simulink model "non_Cascaded_I_PD"  (R2025a)
settings: Solver=VariableStepAuto  StartTime=0.0  StopTime=500  FixedStep=0.01  RelTol=1e-3
InitFcn:
  | parameters
values from neighbouring files (symbols this model uses):
  A = pi*(d/2)^2    (= 0.00321699087728)    [parameters.m]    (also in simulations_code.m = 0.00785398163397; test.m = 0.00785398163397)
  A_cross = 0.090    (= 0.09)    [parameters.m]    (also in simulations_code.m = 0.07; test.m = 0.07)
  C_d = 0.136    [parameters.m]    (also in simulations_code.m = 1; test.m = 1)
  constant_amplitude = 0    [Mission.m]    (also in sensitivity.m)
  d1 = 2    [parameters.m]    (also in simulation_matlab.m = 5; simulations_code.m = 5; test.m = 5)
  F_pos = 0.300 * g + m*g    (= 49.70727)    [parameters.m]    (also in sensitivity.m = 0.300 * g + m_values(i)*g; simulation_matlab.m = 2.94; simulations_code.m = 32.37; test.m = 32.37)
  g = 9.81    [parameters.m]    (also in simulation_matlab.m; simulations_code.m; test.m)
  k_m = 50    [simulation_matlab.m]    (also in simulations_code.m = 5; test.m = 5)
  m = 4.567+0.2    (= 4.767)    [parameters.m]    (also in simulation_matlab.m = 3; simulations_code.m = 3; test.m = 3)
  m_a = 0    [parameters.m]    (also in simulation_matlab.m; simulations_code.m = 2.5; test.m = 2.5)
  p = 0.002    [parameters.m]    (also in simulation_matlab.m; simulations_code.m; test.m)
  rho = 1000    [parameters.m]    (also in simulation_matlab.m; simulations_code.m; test.m)
  sine_amplitude = 0    [Mission.m]    (also in sensitivity.m)
  x_max = V_max / A    (= 0.155424749113)    [parameters.m]    (also in simulations_code.m = 0.0636619772368)
  z_ref = 3    [compare_controllers.m]    (also in simulation_matlab.m = 5; simulations_code.m; test.m; test_scenarios.m = 5)
libraries: slpidlib x1
settings Model: Creator=hannasennero  LastModifiedBy=hannasennero
settings SolverCC: ZeroCrossAlgorithm=Adaptive
settings DebuggingCC: IgnoredZcDiagnostic=none

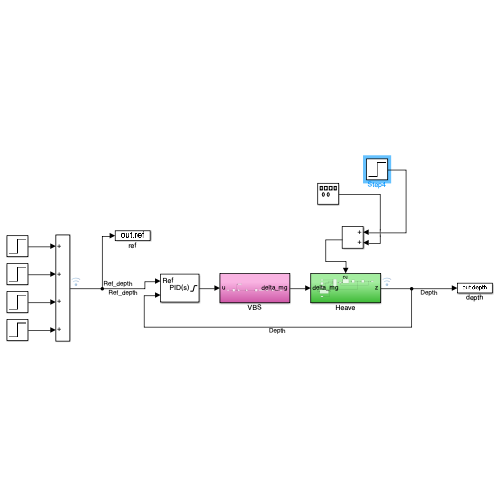
[thumbnail: Simulink's stored preview of the top-level diagram]
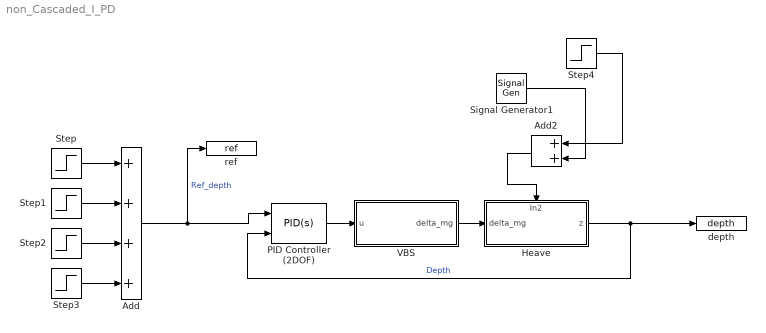
== system non_Cascaded_I_PD ==
  Add : Sum  Inputs=++++
  Add2 : Sum
  Heave : Subsystem
      settings: PortSchema="{\"entries\":[{\"content\":{\"sides\":[{\"content\":{\"connectorIds\":[\"In1\"]},\"type\":\"ConnectorPlacement.EquallySpacedRectSide\",\"uuid\":\"59829fc3-5d95-4f9e-ae89-c400f0704383\"},{\"content\":{\"connectorIds\":[\"Out1\"],\"side\":\"RIGHT\"},\"type\":\"ConnectorPlacement.EquallySpacedRectSide\",\"uuid\":\"26090ad4-c6e5-41d3-8575-8e5c66b7a9e5\"},{\"content\":{\"connectorIds\":[\"In2\"],\"side\":\"TOP\"},\"type\":\"ConnectorPlacement.EquallySpacedRectSide\",\"uuid\":\"d235516f-c242-4726-8776-5975a902e983\"}]},\"type\":\"ConnectorPlacement.EquallySpacedConnector\",\"uuid\":\"fae2b3b8-8546-4969-b5ff-a1ca4f448a21\"}],\"packageUris\":[\"http://schema.mathworks.com/mf0/Connector/R2020b\"],\"version\":\"1.0\"}"
  PID Controller (2DOF) : slpidlib/PID Controller (2DOF)  Controller=PID  Form=Parallel  TimeDomain=Continuous-time  UseExternalTs=off  SampleTime=-1  IntegratorMethod=Forward Euler  FilterMethod=Forward Euler  ControllerParametersSource=internal  P=0.8  I=0.03  UseKiTs=off  D=1  UseExternalDerivativeSource=off  N=1  UseFilter=on  b=0  c=0  TunerSelectOption=Transfer Function Based (PID Tuner App)  InitialConditionSource=internal  InitialConditionForIntegrator=0  InitialConditionForFilter=0  DifferentiatorICPrevScaledInput=0  ExternalReset=none  TrackingMode=off  Kt=1  LimitOutput=on  SatLimitsSource=internal  UpperSaturationLimit=1  LowerSaturationLimit=-1  LinearizeAsGain=on  AntiWindupMode=clamping  Kb=1  LimitIntegrator=off  UpperIntegratorSaturationLimit=inf  LowerIntegratorSaturationLimit=-inf  POutMin=[]  POutMax=[]  IOutMin=[]  IOutMax=[]  DOutMin=[]  DOutMax=[]  NOutMin=[]  NOutMax=[]  bOutMin=[]  bOutMax=[]  cOutMin=[]  cOutMax=[]  SumOutMin=[]  SumOutMax=[]  SaturationOutMin=[]  SaturationOutMax=[]  PParamMin=[]  PParamMax=[]  IParamMin=[]  IParamMax=[]  DParamMin=[]  DParamMax=[]  NParamMin=[]  NParamMax=[]  bParamMin=[]  bParamMax=[]  cParamMin=[]  cParamMax=[]  KbParamMin=[]  KbParamMax=[]  KtParamMin=[]  KtParamMax=[]  KbOutMin=[]  KbOutMax=[]  KtOutMin=[]  KtOutMax=[]  IntegratorOutMin=[]  IntegratorOutMax=[]  FilterOutMin=[]  FilterOutMax=[]  SumI1OutMin=[]  SumI1OutMax=[]  SumI2OutMin=[]  SumI2OutMax=[]  SumI3OutMin=[]  SumI3OutMax=[]  SumI4OutMin=[]  SumI4OutMax=[]  SumDOutMin=[]  SumDOutMax=[]  Sum1OutMin=[]  Sum1OutMax=[]  Sum2OutMin=[]  Sum2OutMax=[]  Sum3OutMin=[]  Sum3OutMax=[]  DifferentiatorOutMin=[]  DifferentiatorOutMax=[]  FilterDiffOutCoefMin=[]  FilterDiffOutCoefMax=[]  ReciprocalOutMin=[]  ReciprocalOutMax=[]  SumDenOutMin=[]  SumDenOutMax=[]  SumNumOutMin=[]  SumNumOutMax=[]  DivideOutMin=[]  DivideOutMax=[]  UdiffTsProdOutMin=[]  UdiffTsProdOutMax=[]  NTsProdOutMin=[]  NTsProdOutMax=[]  UintegralTsProdOutMin=[]  UintegralTsProdOutMax=[]  UngainTsProdOutMin=[]  UngainTsProdOutMax=[]  ClampingZeroOutDataTypeStr=Inherit: Inherit via back propagation  ClampingZeroOutMin=[]  ClampingZeroOutMax=[]  FilterDenConstantOutDataTypeStr=Inherit: Inherit via back propagation  FilterDenConstantOutMin=[]  FilterDenConstantOutMax=[]  PCopyOutDataTypeStr=Inherit: Inherit via back propagation  PCopyOutMin=[]  PCopyOutMax=[]  NCopyOutDataTypeStr=Inherit: Inherit via back propagation  NCopyOutMin=[]  NCopyOutMax=[]  IntegratorContinuousStateAttributes=''  IntegratorStateMustResolveToSignalObject=off  IntegratorRTWStateStorageClass=Auto  FilterContinuousStateAttributes=''  FilterStateMustResolveToSignalObject=off  FilterRTWStateStorageClass=Auto  ParallelPVariant=InternalParameters  IdealPVariant=Disabled  IVariant=InternalParameters  DVariant=InternalParameters  bVariant=InternalParameters  cVariant=InternalParameters  IntegratorVariant=Continuous  SatVariant=Enabled  AWVariant=ContClampingParallel  PCopyVariant=Disabled  TRVariant=Disabled  FdbkBlocksVariant=Forward  IdealPFdbkVariant=Disabled  SatFdbkVariant=Disabled  DerivativeFilterVariant=ContFilter  NVariant=InternalParameters  NCopyVariant=Disabled  FilterICVariant=InternalICsFilter  IntegratorICVariant=InternalICs  ExternalResetVariant=Disabled  TRSumVariant=Passthrough  SumFdbkVariant=Disabled  SumVariant=Sum_PID  TsampFilterVariant=InternalTs  TsampNgainVariant=Passthrough  TsampIntegralVariant=Disabled_SignalSpec  ExternalSaturationOutDataTypeStr=Inherit: Same as second input  DerivativeSourceVariant=ErrorSignal  PreIntVariant=InternalPreInt
  Signal Generator1 : SignalGenerator  Amplitude=sine_amplitude  Frequency=0.05
  Step : Step  After=z_ref  SampleTime=0
  Step1 : Step  Time=100  After=0  SampleTime=0
  Step2 : Step  Time=200  After=0  SampleTime=0
  Step3 : Step  Time=400  After=0  SampleTime=0
  Step4 : Step  Time=40  After=constant_amplitude  SampleTime=0
  VBS : Subsystem
  depth : ToWorkspace  VariableName=depth  SaveFormat=Timeseries  SampleTime=-1
  ref : ToWorkspace  VariableName=ref  SaveFormat=Timeseries  SampleTime=-1
  wires:
  Heave/1(z) -> PID Controller (2DOF)/2, depth/1  "Depth"
  VBS/1(delta_mg) -> Heave/1(delta_mg)
  PID Controller (2DOF)/1 -> VBS/1(u)
  Step1/1 -> Add/2
  Step/1 -> Add/1
  Step2/1 -> Add/3
  Step3/1 -> Add/4
  Add/1 -> ref/1, PID Controller (2DOF)/1  "Ref_depth"
  Signal Generator1/1 -> Add2/2
  Add2/1 -> Heave/2(In2)
  Step4/1 -> Add2/1

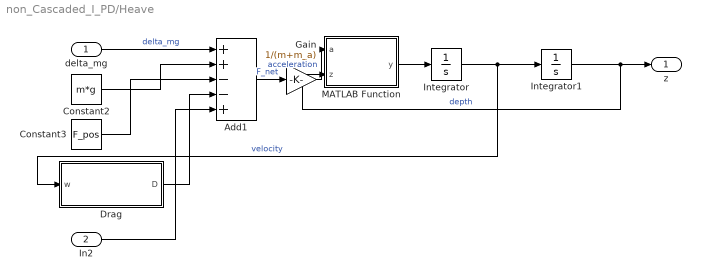
== system non_Cascaded_I_PD/Heave ==
  delta_mg : Inport
  In2 : Inport  Port=2
  Add1 : Sum  Inputs=++--+
  Constant2 : Constant  Value=m*g
  Constant3 : Constant  Value=F_pos
  Drag : Subsystem
  Gain : Gain  Gain=1/(m+m_a)
  Integrator : Integrator  LowerSaturationLimit=0
  Integrator1 : Integrator  LimitOutput=on  LowerSaturationLimit=0
  MATLAB Function : MATLAB Function  TreatAsAtomicUnit=on
  z : Outport
  wires:
  delta_mg/1 -> Add1/1  "delta_mg"
  Constant2/1 -> Add1/2
  Constant3/1 -> Add1/3
  Drag/1(D) -> Add1/4
  Add1/1 -> Gain/1  "F_net"
  Integrator/1 -> Drag/1(w), Integrator1/1  "velocity"
  Integrator1/1 -> MATLAB Function/2(z), z/1  "depth"
  MATLAB Function/1(y) -> Integrator/1
  Gain/1 -> MATLAB Function/1(a)  "acceleration"
  In2/1 -> Add1/5

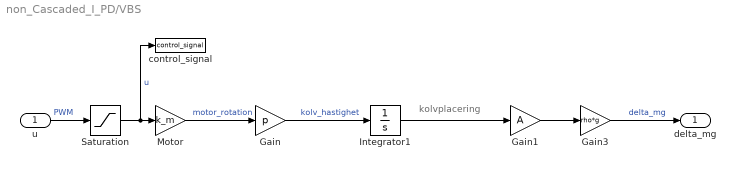
== system non_Cascaded_I_PD/VBS ==
  note: kolvplacering
  u : Inport
  Gain : Gain  Gain=p
  Gain1 : Gain  Gain=A
  Gain3 : Gain  Gain=rho*g
  Integrator1 : Integrator  LimitOutput=on  UpperSaturationLimit=x_max  LowerSaturationLimit=0
  Motor : Gain  Gain=k_m
  Saturation : Saturate  UpperLimit=1  LowerLimit=-1  LinearizeAsGain=off
  control_signal : ToWorkspace  VariableName=control_signal  SaveFormat=Timeseries  SampleTime=-1
  delta_mg : Outport
  wires:
  Motor/1 -> Gain/1  "motor_rotation"
  u/1 -> Saturation/1  "PWM"
  Gain/1 -> Integrator1/1  "kolv_hastighet"
  Integrator1/1 -> Gain1/1
  Gain1/1 -> Gain3/1
  Gain3/1 -> delta_mg/1  "delta_mg"
  Saturation/1 -> control_signal/1, Motor/1  "u"

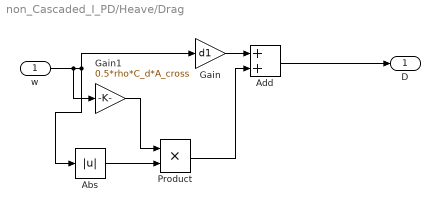
== system non_Cascaded_I_PD/Heave/Drag ==
  w : Inport
  Abs : Abs  SaturateOnIntegerOverflow=off
  Add : Sum
  Gain : Gain  Gain=d1
  Gain1 : Gain  Gain=0.5*rho*C_d*A_cross
  Product : Product
  D : Outport
  wires:
  w/1 -> Gain/1, Abs/1, Gain1/1
  Gain/1 -> Add/1
  Abs/1 -> Product/2
  Gain1/1 -> Product/1
  Product/1 -> Add/2
  Add/1 -> D/1

== matlab function non_Cascaded_I_PD/Heave/MATLAB Function ==
  data: a input; y output; z input
function y = fcn(a,z)
if a<= 0 && z <= 0
    y = 0;
else
    y = a;
end
